simulink model "s0313"  (Simulink 6.0)
settings: Solver=ode3  SolverMode=SingleTasking  StartTime=0.0  StopTime=900  FixedStep=1  MaxStep=1  RelTol=1e-3  AbsTol=1e-6
values from neighbouring files (symbols this model uses):
  T1 = 3*T1    (= 0.3)    [m0203.m]    (also in m0204.m = 0.1; m0205.m = 0.1; m0207.m = 0.1; m0221d.m = 1/a0)
  ydach = 1    [m0305.m]    (also in m0306.m; m0311.m; m0312b.m; m0313.m)
settings Model: LastModifiedBy=Froriep
settings DataIOCC: LimitDataPoints=off  SaveOutput=off  SaveTime=off
settings OptimizationCC: BooleanDataType=off
settings DebuggingCC: SolverPrmCheckMsg=none
settings HardwareCC: TargetUnknown=on
settings GRTTargetCC: ModelReferenceCompliant=off  MatFileLogging=off

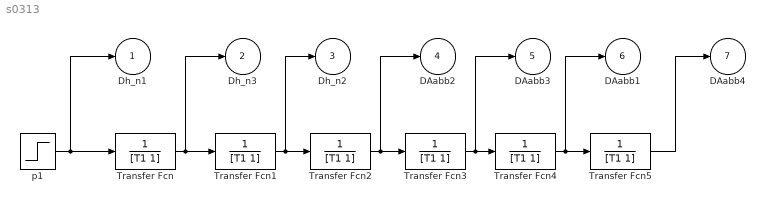
== system s0313 ==
  Transfer Fcn{,1..5} (6 alike) : TransferFcn  Denominator=[T1 1]
  p1 : Step  Time=0  After=ydach  SampleTime=0
  Dh_n1 : Outport
  Dh_n3 : Outport  Port=2
  Dh_n2 : Outport  Port=3
  DAabb2 : Outport  Port=4
  DAabb3 : Outport  Port=5
  DAabb1 : Outport  Port=6
  DAabb4 : Outport  Port=7
  wires:
  Transfer Fcn/1 -> Transfer Fcn1/1, Dh_n3/1
  Transfer Fcn1/1 -> Transfer Fcn2/1, Dh_n2/1
  Transfer Fcn2/1 -> Transfer Fcn3/1, DAabb2/1
  Transfer Fcn3/1 -> Transfer Fcn4/1, DAabb3/1
  Transfer Fcn4/1 -> Transfer Fcn5/1, DAabb1/1
  Transfer Fcn5/1 -> DAabb4/1
  p1/1 -> Transfer Fcn/1, Dh_n1/1
